simulink model "SimulationModel_FLC2"  (R2018a)
settings: Solver=ode4  StartTime=0.0  StopTime=inf  RelTol=1e-3
PreLoadFcn:
  | addLibrariesInPath('sim')
PostLoadFcn:
  | loadRobotParameters
StartFcn:
  | simApp = SimDisplay.getInstance;
  | simApp.reset;
  | simApp.TrackView.setup(double(SitesPositions), ObstaclesPositions,ObstaclesVertices,ObstaclesEdges);
values from neighbouring files (symbols this model uses):
  AngularSpeed = 300    [loadRobotParameters.m]
  AxleLength = 16.7    [loadRobotParameters.m]
  DISTANCE_APPROACH = 45    [loadRobotParameters.m]
  DISTANCE_MAX = 200    [loadRobotParameters.m]
  DISTANCE_PARKING = 10    [loadRobotParameters.m]
  do_one_run = true    [loadRobotParameters.m]
  EncL_init = 0    [loadRobotParameters.m]
  EncR_init = 0    [loadRobotParameters.m]
  EncRes = 636    [loadRobotParameters.m]
  lcam = [21, 90]    [loadRobotParameters.m]
  motorL = [-967.207000 -900.359000 -783.375000 -618.344000 -325.884000 -0.000000 0.000000 325.884000 618.344000 783.375000 900.359000 967.207000 ]    [loadRobotParameters.m]
  motorR = [-937.961000 -850.223000 -768.752000 -618.344000 -302.905000 -0.000000 0.000000 302.905000 618.344000 768.752000 850.223000 937.961000 ]    [loadRobotParameters.m]
  motorX = [-100.000000 -90.000000 -70.000000 -50.000000 -30.000000 -27.000000 27.000000 30.000000 50.000000 70.000000 90.000000 100.000000 ]    [loadRobotParameters.m]
  pcam = [24, 100]    [loadRobotParameters.m]
  RADIUS_TARGET = 5    [loadRobotParameters.m]
  S_ROT = 10    [loadRobotParameters.m]
  SPEED_APPROACH = 15    [loadRobotParameters.m]
  SPEED_BACK = 5    [loadRobotParameters.m]
  SPEED_NORMAL = 30    [loadRobotParameters.m]
  startPos = single([150 150])    [loadRobotParameters.m]
  TauMotor = 0.1    [loadRobotParameters.m]
  TH1 = 5    [loadRobotParameters.m]
  TH2 = 15    [loadRobotParameters.m]
  theta0 = 0    [loadRobotParameters.m]
  Ts = 0.1    [loadRobotParameters.m]
  WAIT_TIME = 4    [loadRobotParameters.m]
  WheelRadius = 7/2    (= 3.5)    [loadRobotParameters.m]
undefined symbols (not defined in the file or in its folder): ObstaclesEdges, ObstaclesVertices, SitesPositions
libraries: simulink_extras x2, simulink x2, Fuzzy_Type2_Lib x1, realtime_pacer_lib x1, cstblocks x1
(part 1 of 2)
CloseFcn:
  | delete(SimDisplay.getInstance());
settings Model: PauseTimes=14  NumberOfSteps=3  ExtModeTrigDuration=2  Creator=gpacitti  LastModifiedBy=root
settings DataIOCC: LimitDataPoints=on  SaveFormat=Array
settings OptimizationCC: BlockReduction=off  BooleanDataType=off  LifeSpan=inf
settings DebuggingCC: SaveWithParameterizedLinksMsg=none  SignalResolutionControl=TryResolveAllWithWarning  ParameterPrecisionLossMsg=none  AllowSymbolicDim=off  SFUnexpectedBacktrackingDiag=warning  SFNoUnconditionalDefaultTransitionDiag=warning  SFExecutionAtInitializationDiag=none
settings HardwareCC: ProdBitPerPointer=32  ProdBitPerSizeT=32  ProdBitPerPtrDiffT=32  ProdLargestAtomicFloat=None  ProdIntDivRoundTo=Undefined  ProdEndianess=Unspecified  ProdWordSize=32  ProdHWDeviceType=32-bit Generic  TargetUnknown=on
settings ModelReferenceCC: PropagateSignalLabelsOutOfModel=off
settings CodeAppCC: StateflowObjectComments=on
settings GRTTargetCC: TargetLangStandard=C89/C90 (ANSI)  GeneratePreprocessorConditionals=Disable all
settings ConfigComp: CovMetricSettings=dw  CovHtmlReporting=on  CovSaveCumulativeToWorkspaceVar=on  CovSaveSingleToWorkspaceVar=on  CovExternalEMLEnable=off  CovSFcnEnable=off
settings ConfigurationSet: Description=SimMechanics 2G

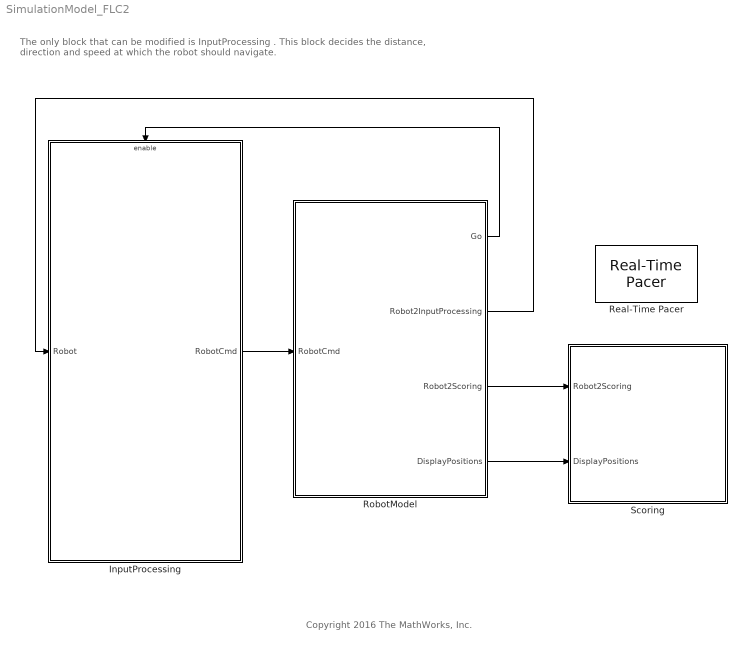
== system SimulationModel_FLC2 ==
  note: Copyright 2016 The MathWorks, Inc.
  note: The only block that can be modified is InputProcessing .
      | This block decides the distance, direction and speed at which the robot should navigate.
  InputProcessing : Subsystem
      mask Display: image('Arduino_Due_2_0274.png',[0.15,0.3,0.45,0.4]);
  Real-Time Pacer : realtime_pacer_lib/Real-Time Pacer  simTimePerRealTime=1
  RobotModel : Subsystem  mask(Robot){}
      mask help:
      | !! DO NOT MODIFY !!
      | Model representing the robot behavior including physical representation and sensors.
      |
      | Version 2.1
      mask Display: image('robot_3d.jpg',[0.4,0.7,0.45,0.25]);
  Scoring : Subsystem  mask(Scoring){}
      mask help:
      | !! DO NOT MODIFY !!
      | Model representing the judge and visualisation.
  wires:
  RobotModel/2(Robot2InputProcessing) -> InputProcessing/1(Robot)
  RobotModel/3(Robot2Scoring) -> Scoring/1(Robot2Scoring)
  RobotModel/1(Go) -> InputProcessing/Enable
  RobotModel/4(DisplayPositions) -> Scoring/2(DisplayPositions)
  InputProcessing/1(RobotCmd) -> RobotModel/1(RobotCmd)

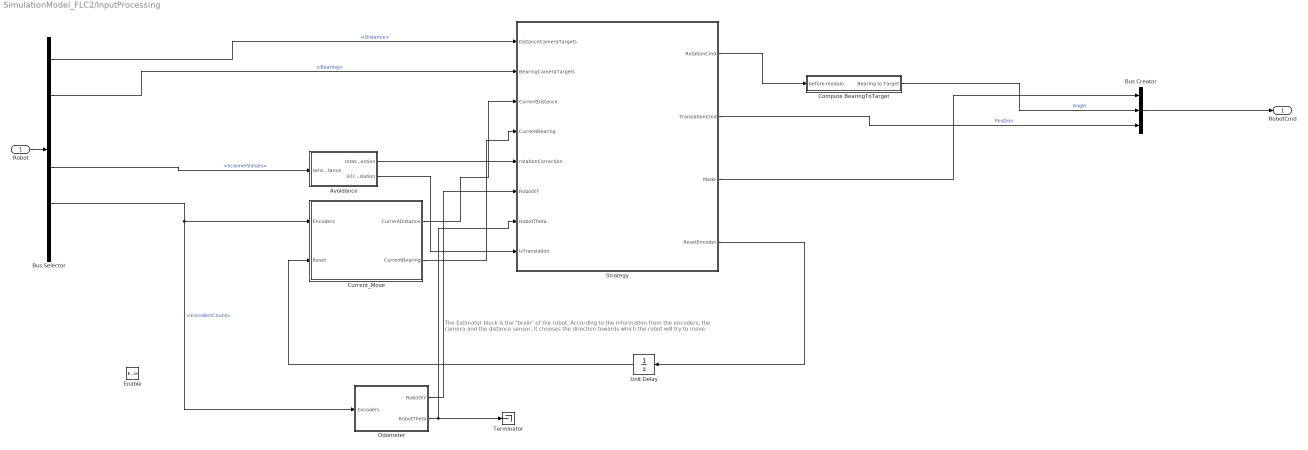
== system SimulationModel_FLC2/InputProcessing ==
  note: The Estimator block is the "brain" of the robot. According to the information from the encoders, the camera and the
      | distance sensor, it chooses the direction towards which the robot will try to move.
  Robot : Inport  OutDataTypeStr=Bus: bus_Robot
  Enable : EnablePort
  Avoidance : Subsystem
  Bus Creator : BusCreator  Inputs=3  OutDataTypeStr=Bus: bus_Command  NonVirtualBus=on
  Bus Selector : BusSelector  OutputSignals=Distance,Bearing,ScannerStatus,ScannerValues,EncodersCount,Remaining
  Compute BearingToTarget : Subsystem
  Current_Move : Subsystem
  Odometer : Subsystem
  Strategy : Stateflow chart  TreatAsAtomicUnit=on
  Terminator : Terminator
  Unit Delay : UnitDelay  SampleTime=-1
  RobotCmd : Outport  OutDataTypeStr=Bus: bus_Command
  wires:
  Robot/1 -> Bus Selector/1
  Bus Selector/2 -> Strategy/2(BearingCameraTargets)  "<Bearing>"
  Bus Selector/4 -> Avoidance/1(sensors distance)  "<ScannerValues>"
  Bus Selector/5 -> Odometer/1(Encoders), Current_Move/1(Encoders)  "<EncodersCount>"
  Bus Selector/1 -> Strategy/1(DistanceCameraTargets)  "<Distance>"
  Strategy/4(ResetEncoder) -> Unit Delay/1
  Unit Delay/1 -> Current_Move/2(Reset)
  Current_Move/1(CurrentDistance) -> Strategy/3(CurrentDistance)
  Odometer/2(RobotTheta) -> Terminator/1, Strategy/7(RobotTheta)
  Odometer/1(RobotXY) -> Strategy/6(RobotXY)
  Current_Move/2(CurrentBearing) -> Strategy/4(CurrentBearing)
  Avoidance/1(rotationCorrection) -> Strategy/5(rotationCorrection)
  Avoidance/2(isTranslation) -> Strategy/8(isTranslation)
  Strategy/1(RotationCmd) -> Compute BearingToTarget/1(before modulo)
  Bus Creator/1 -> RobotCmd/1
  Compute BearingToTarget/1(Bearing to Target) -> Bus Creator/2  "Angle"
  Strategy/2(TranslationCmd) -> Bus Creator/3  "Position"
  Strategy/3(Mode) -> Bus Creator/1

== system SimulationModel_FLC2/RobotModel ==
  RobotCmd : Inport  SampleTime=0
  Bus Creator : BusCreator  Inputs=6  OutDataTypeStr=Bus: bus_Robot  NonVirtualBus=on
  Controller : Subsystem
  Robot : Subsystem
  estimate_position : Subsystem
  Go : Outport
  Robot2InputProcessing : Outport  Port=2  OutDataTypeStr=Bus: bus_Robot
  Robot2Scoring : Outport  Port=3
  DisplayPositions : Outport  Port=4
  wires:
  Robot/6(Go) -> Go/1
  Robot/7(Robot2Scoring) -> Robot2Scoring/1
  Robot/5(ScannerValues) -> Bus Creator/5
  Robot/4(ScannerStatus) -> Bus Creator/4
  Robot/3(Bearing) -> Bus Creator/3
  Robot/2(Distance) -> Bus Creator/2
  Controller/1(MotorDemand) -> Robot/1(MotorDemand)
  Robot/1(EncoderCount) -> Bus Creator/1, estimate_position/1(Encoders), Controller/1(Encoders)
  estimate_position/1(RobotXY) -> DisplayPositions/1
  Controller/2(RemainingAngleDistance) -> Bus Creator/6  "Remaining"
  RobotCmd/1 -> Controller/2(RobotCmd)
  Bus Creator/1 -> Robot2InputProcessing/1  "Robot"

== system SimulationModel_FLC2/Scoring ==
  Robot2Scoring : Inport
  DisplayPositions : Inport  Port=2
  Bus Selector : BusSelector  OutputSignals=Position,Go
  Bus Selector1 : BusSelector  OutputSignals=LocatedTargets,RobotAngle,ArmAngleEstimated
  FigureOutput : Subsystem  TreatAsAtomicUnit=on  SimViewingDevice=on
  Referee : Subsystem
      mask Display: % image(imread('referee.png'))
  wires:
  Referee/1(Targets Located) -> FigureOutput/2(Targets Found)  "TargetsLocated"
  Referee/2(Time Last Target Found) -> FigureOutput/3(Time Last Found)  "TimeLastTargetFound"
  Referee/3(Elapsed Time_sec) -> FigureOutput/4(Time Elapsed)  "ElapsedTime"
  DisplayPositions/1 -> FigureOutput/9(DisplayPositions)
  Robot2Scoring/1 -> Bus Selector1/1, Bus Selector/1
  Bus Selector/2 -> Referee/2(Start Flag)  "<Go>"
  Bus Selector/1 -> FigureOutput/1(Position), Referee/1(Robot Position_m)  "<Position>"
  Bus Selector1/1 -> FigureOutput/5(locatedTargets)  "<LocatedTargets>"
  Bus Selector1/2 -> FigureOutput/6(robottheta)  "<RobotAngle>"
  Bus Selector1/3 -> FigureOutput/8(ArmAngleCommand), FigureOutput/7(ArmAngleEstimated)  "<ArmAngleEstimated>"

== system SimulationModel_FLC2/InputProcessing/Avoidance ==
  sensors distance : Inport
  Constant : Constant  Value=85
  Demux : Demux  Outputs=3
  Demux1 : Demux  Outputs=2
  Interval Type-2 Fuzzy Logic Controller with TR selection : Fuzzy_Type2_Lib/Interval Type-2 Fuzzy Logic Controller with TR selection  t2fisSim=t2fis_Avoidance  TRtype=0
      settings: SourceProductName=Interval Type-2 Fuzzy Logic Systems Toolbox
  Mux : Mux  Inputs=5
  Switch : Switch  Criteria=u2 > Threshold  Threshold=-1
  To File : ToFile  Filename=Avoidance.mat  MatrixName=Avoid
  rotationCorrection : Outport
  isTranslation : Outport  Port=2
  wires:
  Demux1/1 -> Mux/1, rotationCorrection/1  "rot"
  Demux1/2 -> Mux/2, isTranslation/1  "tran"
  Switch/1 -> Interval Type-2 Fuzzy Logic Controller with TR selection/1, Demux/1
  Constant/1 -> Switch/3
  sensors distance/1 -> Switch/2, Switch/1
  Mux/1 -> To File/1
  Demux/1 -> Mux/3
  Demux/2 -> Mux/4
  Demux/3 -> Mux/5
  Interval Type-2 Fuzzy Logic Controller with TR selection/1 -> Demux1/1

== system SimulationModel_FLC2/InputProcessing/Compute BearingToTarget ==
  before modulo : Inport
  Constant : Constant  Value=180  OutDataTypeStr=Inherit: Inherit via back propagation
  Constant1 : Constant  Value=360  OutDataTypeStr=Inherit: Inherit via back propagation
  Math Function1 : Math  Operator=mod  SaturateOnIntegerOverflow=on
  Sum10 : Sum  Inputs=-+|
  Sum7 : Sum  Inputs=++|
  Bearing to Target : Outport  SampleTime=Ts
  wires:
  Constant/1 -> Sum7/1, Sum10/1
  Sum7/1 -> Math Function1/1
  Constant1/1 -> Math Function1/2
  Math Function1/1 -> Sum10/2
  Sum10/1 -> Bearing to Target/1
  before modulo/1 -> Sum7/2

== system SimulationModel_FLC2/InputProcessing/Current_Move ==
  Encoders : Inport
  Reset : Inport  Port=2
  Add : Sum
  Add1 : Sum  Inputs=-+
  Demux : Demux  Outputs=2
  Gain : Gain  Gain=1/2
  Gain1 : Gain  Gain=180/(AxleLength*pi)
  d : Subsystem
  CurrentDistance : Outport
  CurrentBearing : Outport  Port=2
  wires:
  Reset/1 -> d/2(reset)
  Demux/2 -> Add/2, Add1/2
  Add1/1 -> Gain1/1
  Gain1/1 -> CurrentBearing/1
  Gain/1 -> CurrentDistance/1
  Demux/1 -> Add1/1, Add/1
  Add/1 -> Gain/1
  Encoders/1 -> d/1(encoder)
  d/1(d) -> Demux/1

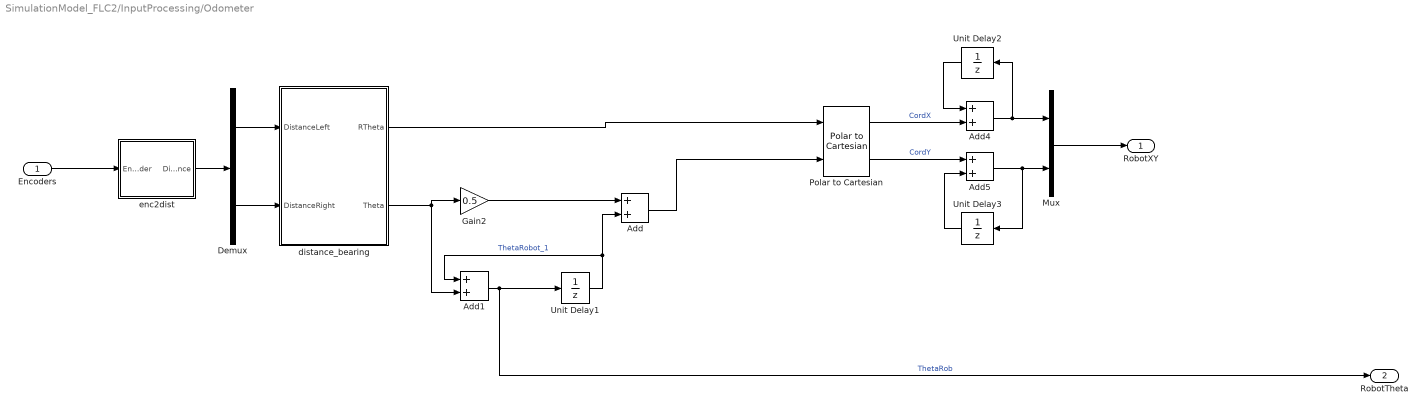
== system SimulationModel_FLC2/InputProcessing/Odometer ==
  Encoders : Inport
  Add{,1,4..5} (4 alike) : Sum
  Demux : Demux  Outputs=2
  Gain2 : Gain  Gain=0.5
  Mux : Mux  Inputs=2
  Polar to Cartesian : simulink_extras/Transformations/Polar to Cartesian
      settings: SourceProductName=Simulink  SourceProductBaseCode=SL
  Unit Delay1 : UnitDelay  DialogController=Simulink.DDGSource  InitialCondition=theta0*pi/180  SampleTime=-1
  Unit Delay2 : UnitDelay  DialogController=Simulink.DDGSource  InitialCondition=single(startPos(1))  SampleTime=-1
  Unit Delay3 : UnitDelay  DialogController=Simulink.DDGSource  InitialCondition=single(startPos(2))  SampleTime=-1
  distance_bearing : Subsystem
  enc2dist : Subsystem
  RobotXY : Outport
  RobotTheta : Outport  Port=2
  wires:
  Gain2/1 -> Add/1
  Polar to Cartesian/1 -> Add4/2  "CordX"
  Polar to Cartesian/2 -> Add5/1  "CordY"
  Add4/1 -> Unit Delay2/1, Mux/1
  Unit Delay2/1 -> Add4/1
  Add5/1 -> Mux/2, Unit Delay3/1
  Unit Delay3/1 -> Add5/2
  distance_bearing/2(Theta) -> Gain2/1, Add1/2
  Unit Delay1/1 -> Add1/1, Add/2  "ThetaRobot_1"
  Add/1 -> Polar to Cartesian/2
  Add1/1 -> RobotTheta/1, Unit Delay1/1  "ThetaRob"
  distance_bearing/1(RTheta) -> Polar to Cartesian/1
  Mux/1 -> RobotXY/1
  enc2dist/1(Distance) -> Demux/1
  Demux/1 -> distance_bearing/1(DistanceLeft)
  Demux/2 -> distance_bearing/2(DistanceRight)
  Encoders/1 -> enc2dist/1(Encoder)

== system SimulationModel_FLC2/RobotModel/Controller ==
  Encoders : Inport
  RobotCmd : Inport  Port=2  OutDataTypeStr=Bus: bus_Command
  Command2Demand : Subsystem
  FeedbackController : Subsystem  VariantControl=variantBasic
  MotorDemand : Outport  SampleTime=Ts  OutputWhenDisabled=reset  InitialOutput=0
  RemainingAngleDistance : Outport  Port=2  OutputWhenDisabled=reset  InitialOutput=0
  wires:
  FeedbackController/3(RemainingAngleDistance) -> RemainingAngleDistance/1
  FeedbackController/1(DifferentialCommand) -> Command2Demand/1(DifferentialCommand)
  FeedbackController/2(ForwardCommand) -> Command2Demand/2(ForwardCommand)
  Command2Demand/1(MotorDemand) -> MotorDemand/1
  Encoders/1 -> FeedbackController/1(Encoders)
  RobotCmd/1 -> FeedbackController/2(Cmd)

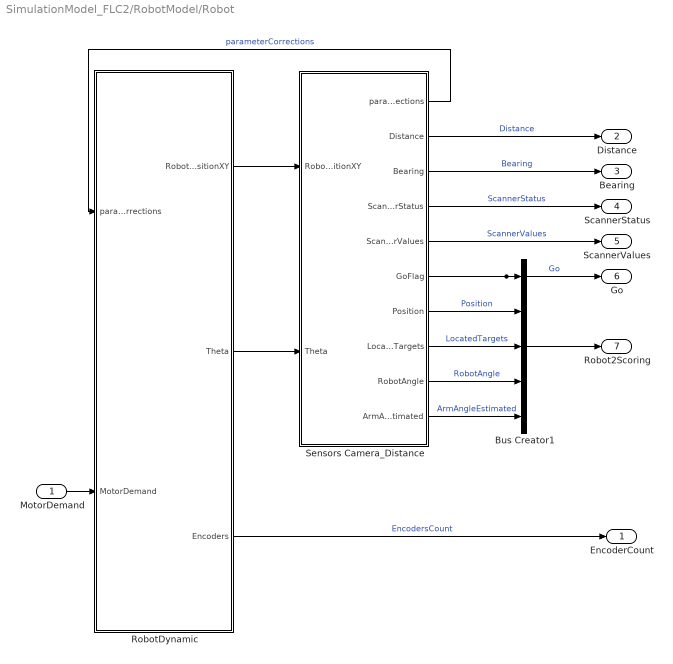
== system SimulationModel_FLC2/RobotModel/Robot ==
  MotorDemand : Inport
  Bus Creator1 : BusCreator  Inputs=5
  RobotDynamic : Subsystem
  Sensors Camera_Distance : Subsystem
  EncoderCount : Outport
  Distance : Outport  Port=2
  Bearing : Outport  Port=3
  ScannerStatus : Outport  Port=4
  ScannerValues : Outport  Port=5
  Go : Outport  Port=6
  Robot2Scoring : Outport  Port=7
  wires:
  Bus Creator1/1 -> Robot2Scoring/1
  Sensors Camera_Distance/10(ArmAngleEstimated) -> Bus Creator1/5  "ArmAngleEstimated"
  Sensors Camera_Distance/9(RobotAngle) -> Bus Creator1/4  "RobotAngle"
  Sensors Camera_Distance/7(Position) -> Bus Creator1/2  "Position"
  Sensors Camera_Distance/8(LocatedTargets) -> Bus Creator1/3  "LocatedTargets"
  MotorDemand/1 -> RobotDynamic/2(MotorDemand)
  Sensors Camera_Distance/6(GoFlag) -> Go/1, Bus Creator1/1  "Go"
  Sensors Camera_Distance/1(parameterCorrections) -> RobotDynamic/1(parameterCorrections)  "parameterCorrections"
  Sensors Camera_Distance/2(Distance) -> Distance/1  "Distance"
  Sensors Camera_Distance/3(Bearing) -> Bearing/1  "Bearing"
  Sensors Camera_Distance/4(ScannerStatus) -> ScannerStatus/1  "ScannerStatus"
  Sensors Camera_Distance/5(ScannerValues) -> ScannerValues/1  "ScannerValues"
  RobotDynamic/3(Encoders) -> EncoderCount/1  "EncodersCount"
  RobotDynamic/1(RobotPositionXY) -> Sensors Camera_Distance/1(RobotPositionXY)
  RobotDynamic/2(Theta) -> Sensors Camera_Distance/2(Theta)

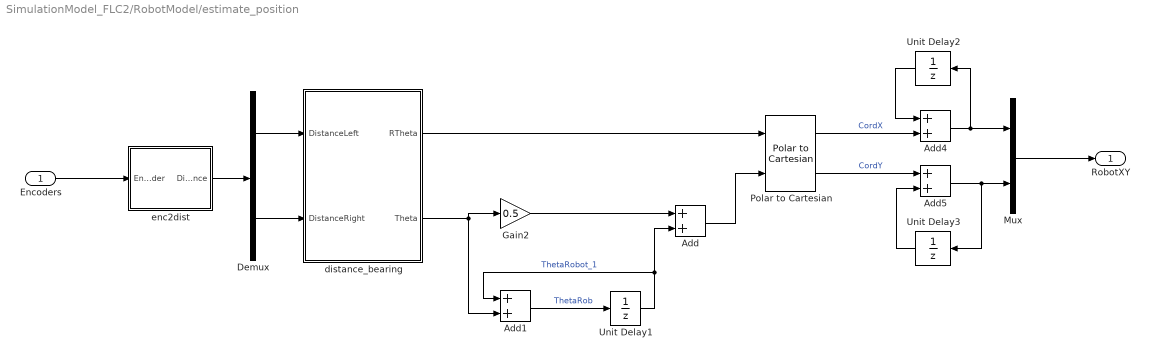
== system SimulationModel_FLC2/RobotModel/estimate_position ==
  Encoders : Inport
  Add{,1,4..5} (4 alike) : Sum
  Demux : Demux  Outputs=2
  Gain2 : Gain  Gain=0.5
  Mux : Mux  Inputs=2
  Polar to Cartesian : simulink_extras/Transformations/Polar to Cartesian
      settings: SourceProductName=Simulink  SourceProductBaseCode=SL
  Unit Delay1 : UnitDelay  DialogController=Simulink.DDGSource  InitialCondition=theta0*pi/180  SampleTime=-1
  Unit Delay2 : UnitDelay  DialogController=Simulink.DDGSource  InitialCondition=single(startPos(1))  SampleTime=-1
  Unit Delay3 : UnitDelay  DialogController=Simulink.DDGSource  InitialCondition=single(startPos(2))  SampleTime=-1
  distance_bearing : Subsystem
  enc2dist : Subsystem
  RobotXY : Outport
  wires:
  Encoders/1 -> enc2dist/1(Encoder)
  Demux/2 -> distance_bearing/2(DistanceRight)
  Demux/1 -> distance_bearing/1(DistanceLeft)
  enc2dist/1(Distance) -> Demux/1
  Mux/1 -> RobotXY/1
  distance_bearing/1(RTheta) -> Polar to Cartesian/1
  Add1/1 -> Unit Delay1/1  "ThetaRob"
  Add/1 -> Polar to Cartesian/2
  Unit Delay1/1 -> Add/2, Add1/1  "ThetaRobot_1"
  distance_bearing/2(Theta) -> Add1/2, Gain2/1
  Unit Delay3/1 -> Add5/2
  Add5/1 -> Unit Delay3/1, Mux/2
  Unit Delay2/1 -> Add4/1
  Add4/1 -> Mux/1, Unit Delay2/1
  Polar to Cartesian/2 -> Add5/1  "CordY"
  Polar to Cartesian/1 -> Add4/2  "CordX"
  Gain2/1 -> Add/1

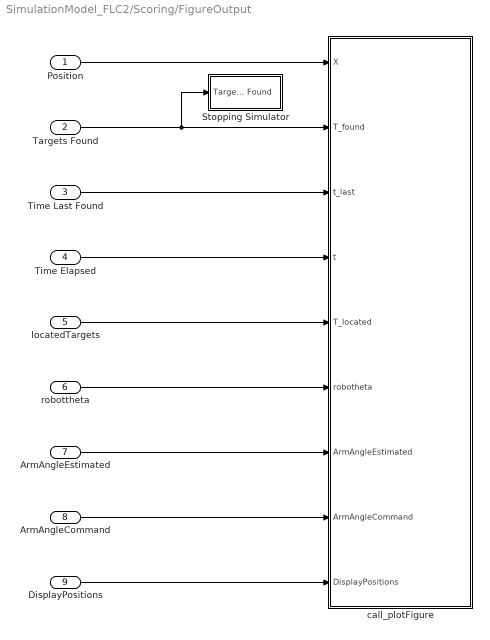
== system SimulationModel_FLC2/Scoring/FigureOutput ==
  Position : Inport
  Targets Found : Inport  Port=2
  Time Last Found : Inport  Port=3
  Time Elapsed : Inport  Port=4
  locatedTargets : Inport  Port=5
  robottheta : Inport  Port=6
  ArmAngleEstimated : Inport  Port=7
  ArmAngleCommand : Inport  Port=8
  DisplayPositions : Inport  Port=9
  Stopping Simulator : Subsystem
  call_plotFigure : MATLAB Function  TreatAsAtomicUnit=on
  wires:
  Position/1 -> call_plotFigure/1(X)
  Targets Found/1 -> Stopping Simulator/1(Targets Found), call_plotFigure/2(T_found)
  Time Last Found/1 -> call_plotFigure/3(t_last)
  Time Elapsed/1 -> call_plotFigure/4(t)
  locatedTargets/1 -> call_plotFigure/5(T_located)
  robottheta/1 -> call_plotFigure/6(robotheta)
  DisplayPositions/1 -> call_plotFigure/9(DisplayPositions)
  ArmAngleEstimated/1 -> call_plotFigure/7(ArmAngleEstimated)
  ArmAngleCommand/1 -> call_plotFigure/8(ArmAngleCommand)

== system SimulationModel_FLC2/Scoring/Referee ==
  Robot Position_m : Inport  SampleTime=Ts
  Start Flag : Inport  Port=2  OutDataTypeStr=boolean  SampleTime=Ts
  Digital Clock1 : DigitalClock  SampleTime=Ts
  Referee : Stateflow chart  TreatAsAtomicUnit=on
  Reshape : Reshape  OutputDimensionality=Row vector (2-D)
  Targets Located : Outport
  Time Last Target Found : Outport  Port=2  PortDimensions=1
  Elapsed Time_sec : Outport  Port=3  PortDimensions=1
  wires:
  Referee/1(timeLastTargetFound) -> Time Last Target Found/1
  Referee/3(targetsFound) -> Targets Located/1
  Robot Position_m/1 -> Reshape/1
  Start Flag/1 -> Referee/2(StartFlag)
  Reshape/1 -> Referee/1(robotPosition)
  Referee/2(elapsedTime) -> Elapsed Time_sec/1
  Digital Clock1/1 -> Referee/3(sim_time)

== system SimulationModel_FLC2/InputProcessing/Current_Move/d ==
  encoder : Inport
  reset : Inport  Port=2
  Add : Sum  Inputs=-+  OutDataTypeStr=single
  Gain : Gain  Gain=2*pi/EncRes
  Product : Product
  Triggered Subsystem : Subsystem  TreatAsAtomicUnit=on
  WheelRadius : Constant  Value=WheelRadius  OutDataTypeStr=Inherit: Inherit via back propagation
  d : Outport
  wires:
  Triggered Subsystem/1(encoderTarget) -> Add/1
  reset/1 -> Triggered Subsystem/Trigger
  encoder/1 -> Triggered Subsystem/1(encoderIn), Add/2
  Gain/1 -> d/1
  Add/1 -> Product/2
  Product/1 -> Gain/1
  WheelRadius/1 -> Product/1

== system SimulationModel_FLC2/InputProcessing/Odometer/distance_bearing ==
  DistanceLeft : Inport
  DistanceRight : Inport  Port=2
  Add : Sum
  Add1 : Sum  Inputs=-+
  Gain : Gain  Gain=0.5
  Gain1 : Gain  Gain=1/AxleLength
  RTheta : Outport
  Theta : Outport  Port=2
  wires:
  Gain1/1 -> Theta/1
  Add/1 -> Gain/1
  Gain/1 -> RTheta/1
  Add1/1 -> Gain1/1
  DistanceLeft/1 -> Add1/1, Add/1
  DistanceRight/1 -> Add/2, Add1/2

== system SimulationModel_FLC2/InputProcessing/Odometer/enc2dist ==
  Encoder : Inport
  Add2 : Sum  Inputs=-+
  Gain : Gain  Gain=2*pi/EncRes  OutDataTypeStr=single
  Product : Product
  Unit Delay : UnitDelay  DialogController=Simulink.DDGSource  SampleTime=-1
  WheelRadius : Constant  Value=WheelRadius  OutDataTypeStr=single
  Distance : Outport
  wires:
  Product/1 -> Gain/1
  Encoder/1 -> Product/1
  Gain/1 -> Unit Delay/1, Add2/2
  Unit Delay/1 -> Add2/1
  Add2/1 -> Distance/1
  WheelRadius/1 -> Product/2

== system SimulationModel_FLC2/RobotModel/Controller/Command2Demand ==
  DifferentialCommand : Inport
  ForwardCommand : Inport  Port=2
  Mux : Mux  Inputs=2
  Saturation : Saturate  UpperLimit=100  LowerLimit=-100
  Saturation1 : Saturate  UpperLimit=100  LowerLimit=-100
  Sum : Sum  Inputs=|++
  Sum1 : Sum  Inputs=-+|
  MotorDemand : Outport
  wires:
  Mux/1 -> MotorDemand/1
  Saturation1/1 -> Mux/2  "RightMotorDemand"
  Saturation/1 -> Mux/1  "LeftMotorDemand"
  Sum1/1 -> Saturation1/1
  Sum/1 -> Saturation/1
  ForwardCommand/1 -> Sum/1, Sum1/2  "ForwardCommand"
  DifferentialCommand/1 -> Sum/2, Sum1/1  "DifferentialCommand"

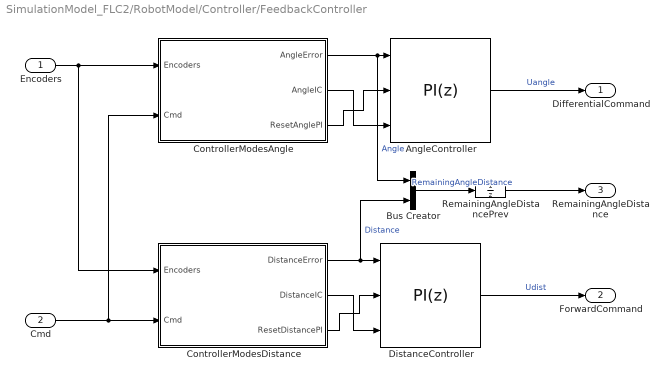
== system SimulationModel_FLC2/RobotModel/Controller/FeedbackController ==
  Encoders : Inport
  Cmd : Inport  Port=2  OutDataTypeStr=Bus: bus_Command
  AngleController : simulink/Continuous/PID Controller  Controller=PI  TimeDomain=Discrete-time  SampleTime=Ts  IntegratorMethod=Forward Euler  FilterMethod=Forward Euler  Form=Parallel  UseFilter=on  ControllerParametersSource=internal  P=1.5  I=1.5  D=1.77054210521092  N=39.6000406506001  InitialConditionSource=external  InitialConditionForIntegrator=0  InitialConditionForFilter=0  ExternalReset=either  LimitOutput=on  UpperSaturationLimit=100  LowerSaturationLimit=-100  LinearizeAsGain=off  AntiWindupMode=clamping  Kb=1  TrackingMode=off  Kt=1  PParamMin=[]  PParamMax=[]  IParamMin=[]  IParamMax=[]  DParamMin=[]  DParamMax=[]  NParamMin=[]  NParamMax=[]  KbParamMin=[]  KbParamMax=[]  KtParamMin=[]  KtParamMax=[]  POutMin=[]  POutMax=[]  IOutMin=[]  IOutMax=[]  DOutMin=[]  DOutMax=[]  NOutMin=[]  NOutMax=[]  KbOutMin=[]  KbOutMax=[]  KtOutMin=[]  KtOutMax=[]  IntegratorOutMin=[]  IntegratorOutMax=[]  FilterOutMin=[]  FilterOutMax=[]  SumOutMin=[]  SumOutMax=[]  SumI1OutMin=[]  SumI1OutMax=[]  SumI2OutMin=[]  SumI2OutMax=[]  SumI3OutMin=[]  SumI3OutMax=[]  SumDOutMin=[]  SumDOutMax=[]  SaturationOutMin=[]  SaturationOutMax=[]  IntegratorContinuousStateAttributes=''  IntegratorStateMustResolveToSignalObject=off  IntegratorRTWStateStorageClass=Auto  FilterContinuousStateAttributes=''  FilterStateMustResolveToSignalObject=off  FilterRTWStateStorageClass=Auto  DifferentiatorICPrevScaledInput=0  DifferentiatorOutMin=[]  DifferentiatorOutMax=[]  FilterDiffOutCoefMin=[]  FilterDiffOutCoefMax=[]  SumDenOutMin=[]  SumDenOutMax=[]  SumNumOutMin=[]  SumNumOutMax=[]  ReciprocalOutMin=[]  ReciprocalOutMax=[]  DivideOutMin=[]  DivideOutMax=[]  TunerSelectOption=Transfer Function Based (PID Tuner App)
  Bus Creator : BusCreator  Inputs=2  OutDataTypeStr=Bus: bus_RemainingPosition  NonVirtualBus=on
  ControllerModesAngle : Stateflow chart  TreatAsAtomicUnit=on
  ControllerModesDistance : Stateflow chart  TreatAsAtomicUnit=on
  DistanceController : simulink/Continuous/PID Controller  Controller=PI  TimeDomain=Discrete-time  SampleTime=Ts  IntegratorMethod=Forward Euler  FilterMethod=Forward Euler  Form=Parallel  UseFilter=on  ControllerParametersSource=internal  P=1.2  I=0.6  D=-10.1274478197245  N=40.1053905161445  InitialConditionSource=external  InitialConditionForIntegrator=0  InitialConditionForFilter=0  ExternalReset=either  LimitOutput=on  UpperSaturationLimit=80  LowerSaturationLimit=-80  LinearizeAsGain=off  AntiWindupMode=clamping  Kb=1  TrackingMode=off  Kt=1  PParamMin=[]  PParamMax=[]  IParamMin=[]  IParamMax=[]  DParamMin=[]  DParamMax=[]  NParamMin=[]  NParamMax=[]  KbParamMin=[]  KbParamMax=[]  KtParamMin=[]  KtParamMax=[]  POutMin=[]  POutMax=[]  IOutMin=[]  IOutMax=[]  DOutMin=[]  DOutMax=[]  NOutMin=[]  NOutMax=[]  KbOutMin=[]  KbOutMax=[]  KtOutMin=[]  KtOutMax=[]  IntegratorOutMin=[]  IntegratorOutMax=[]  FilterOutMin=[]  FilterOutMax=[]  SumOutMin=[]  SumOutMax=[]  SumI1OutMin=[]  SumI1OutMax=[]  SumI2OutMin=[]  SumI2OutMax=[]  SumI3OutMin=[]  SumI3OutMax=[]  SumDOutMin=[]  SumDOutMax=[]  SaturationOutMin=[]  SaturationOutMax=[]  IntegratorContinuousStateAttributes=''  IntegratorStateMustResolveToSignalObject=off  IntegratorRTWStateStorageClass=Auto  FilterContinuousStateAttributes=''  FilterStateMustResolveToSignalObject=off  FilterRTWStateStorageClass=Auto  DifferentiatorICPrevScaledInput=0  DifferentiatorOutMin=[]  DifferentiatorOutMax=[]  FilterDiffOutCoefMin=[]  FilterDiffOutCoefMax=[]  SumDenOutMin=[]  SumDenOutMax=[]  SumNumOutMin=[]  SumNumOutMax=[]  ReciprocalOutMin=[]  ReciprocalOutMax=[]  DivideOutMin=[]  DivideOutMax=[]  TunerSelectOption=Transfer Function Based (PID Tuner App)
  RemainingAngleDistancePrev : UnitDelay  SampleTime=-1
  DifferentialCommand : Outport
  ForwardCommand : Outport  Port=2
  RemainingAngleDistance : Outport  Port=3  OutDataTypeStr=Bus: bus_RemainingPosition
  wires:
  ControllerModesAngle/1(AngleError) -> AngleController/1, Bus Creator/1  "Angle"
  ControllerModesDistance/3(ResetDistancePI) -> DistanceController/2
  ControllerModesDistance/2(DistanceIC) -> DistanceController/3
  ControllerModesDistance/1(DistanceError) -> DistanceController/1, Bus Creator/2  "Distance"
  ControllerModesAngle/3(ResetAnglePI) -> AngleController/2
  ControllerModesAngle/2(AngleIC) -> AngleController/3
  AngleController/1 -> DifferentialCommand/1  "Uangle"
  RemainingAngleDistancePrev/1 -> RemainingAngleDistance/1
  Bus Creator/1 -> RemainingAngleDistancePrev/1  "RemainingAngleDistance"
  Cmd/1 -> ControllerModesDistance/2(Cmd), ControllerModesAngle/2(Cmd)
  Encoders/1 -> ControllerModesDistance/1(Encoders), ControllerModesAngle/1(Encoders)
  DistanceController/1 -> ForwardCommand/1  "Udist"

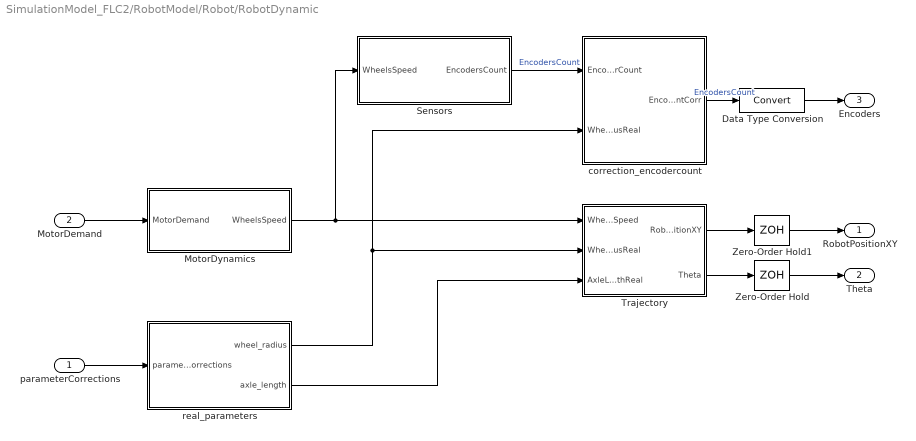
== system SimulationModel_FLC2/RobotModel/Robot/RobotDynamic ==
  parameterCorrections : Inport
  MotorDemand : Inport  Port=2
  Data Type Conversion : DataTypeConversion
  MotorDynamics : Subsystem
  Sensors : Subsystem
  Trajectory : Subsystem
  Zero-Order Hold : ZeroOrderHold  SampleTime=Ts
  Zero-Order Hold1 : ZeroOrderHold  SampleTime=Ts
  correction_encodercount : Subsystem
  real_parameters : Subsystem
  RobotPositionXY : Outport
  Theta : Outport  Port=2
  Encoders : Outport  Port=3
  wires:
  Data Type Conversion/1 -> Encoders/1
  real_parameters/1(wheel_radius) -> correction_encodercount/2(WheelRadiusReal), Trajectory/2(WheelsRadiusReal)
  real_parameters/2(axle_length) -> Trajectory/3(AxleLengthReal)
  Sensors/1(EncodersCount) -> correction_encodercount/1(EncoderCount)  "EncodersCount"
  parameterCorrections/1 -> real_parameters/1(parameterCorrections)
  Zero-Order Hold/1 -> Theta/1
  Zero-Order Hold1/1 -> RobotPositionXY/1
  Trajectory/2(Theta) -> Zero-Order Hold/1
  Trajectory/1(RobotPositionXY) -> Zero-Order Hold1/1
  correction_encodercount/1(EncoderCountCorr) -> Data Type Conversion/1  "EncodersCount"
  MotorDemand/1 -> MotorDynamics/1(MotorDemand)
  MotorDynamics/1(WheelsSpeed) -> Trajectory/1(WheelsSpeed), Sensors/1(WheelsSpeed)

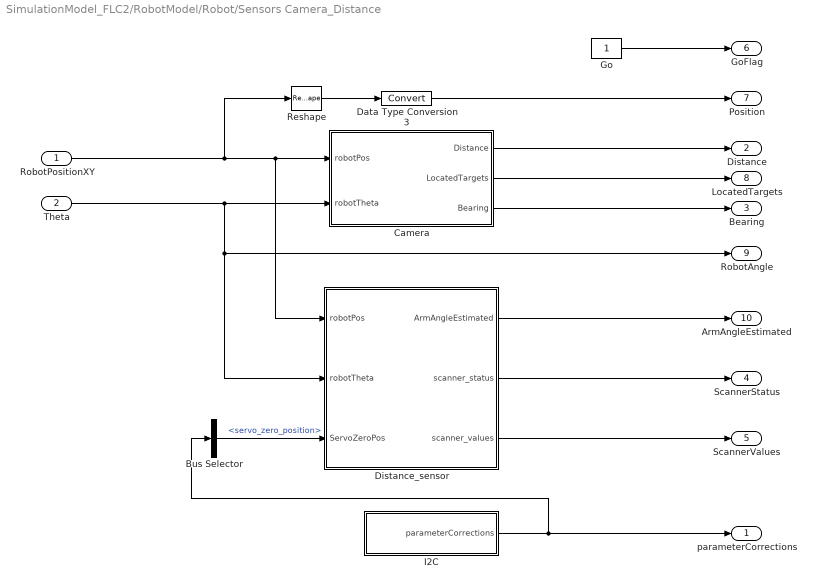
== system SimulationModel_FLC2/RobotModel/Robot/Sensors Camera_Distance ==
  RobotPositionXY : Inport
  Theta : Inport  Port=2
  Bus Selector : BusSelector  OutputSignals=servo_zero_position
  Camera : Subsystem
  Data Type Conversion3 : DataTypeConversion
  Distance_sensor : Subsystem
  Go : Constant  OutMin=0  OutMax=1  OutDataTypeStr=boolean  SampleTime=0.1
  I2C : Subsystem
  Reshape : Reshape  OutputDimensionality=Row vector (2-D)
  parameterCorrections : Outport
  Distance : Outport  Port=2  OutDataTypeStr=int16
  Bearing : Outport  Port=3  OutDataTypeStr=int8
  ScannerStatus : Outport  Port=4
  ScannerValues : Outport  Port=5
  GoFlag : Outport  Port=6
  Position : Outport  Port=7
  LocatedTargets : Outport  Port=8
  RobotAngle : Outport  Port=9
  ArmAngleEstimated : Outport  Port=10
  wires:
  Go/1 -> GoFlag/1
  Bus Selector/1 -> Distance_sensor/3(ServoZeroPos)  "<servo_zero_position>"
  I2C/1(parameterCorrections) -> parameterCorrections/1, Bus Selector/1
  Distance_sensor/3(scanner_values) -> ScannerValues/1
  Distance_sensor/2(scanner_status) -> ScannerStatus/1
  Distance_sensor/1(ArmAngleEstimated) -> ArmAngleEstimated/1
  Camera/3(Bearing) -> Bearing/1
  Camera/2(LocatedTargets) -> LocatedTargets/1
  Camera/1(Distance) -> Distance/1
  Theta/1 -> Camera/2(robotTheta), Distance_sensor/2(robotTheta), RobotAngle/1
  RobotPositionXY/1 -> Reshape/1, Camera/1(robotPos), Distance_sensor/1(robotPos)
  Reshape/1 -> Data Type Conversion3/1
  Data Type Conversion3/1 -> Position/1

== system SimulationModel_FLC2/RobotModel/estimate_position/distance_bearing ==
  DistanceLeft : Inport
  DistanceRight : Inport  Port=2
  Add : Sum
  Add1 : Sum  Inputs=-+
  Gain : Gain  Gain=0.5
  Gain1 : Gain  Gain=1/AxleLength
  RTheta : Outport
  Theta : Outport  Port=2
  wires:
  DistanceRight/1 -> Add1/2, Add/2
  DistanceLeft/1 -> Add/1, Add1/1
  Add1/1 -> Gain1/1
  Gain/1 -> RTheta/1
  Add/1 -> Gain/1
  Gain1/1 -> Theta/1

== system SimulationModel_FLC2/RobotModel/estimate_position/enc2dist ==
  Encoder : Inport
  Add2 : Sum  Inputs=-+
  Gain : Gain  Gain=2*pi/EncRes  OutDataTypeStr=single
  Product : Product
  Unit Delay : UnitDelay  DialogController=Simulink.DDGSource  SampleTime=-1
  WheelRadius : Constant  Value=WheelRadius  OutDataTypeStr=single
  Distance : Outport
  wires:
  WheelRadius/1 -> Product/2
  Add2/1 -> Distance/1
  Unit Delay/1 -> Add2/1
  Gain/1 -> Add2/2, Unit Delay/1
  Encoder/1 -> Product/1
  Product/1 -> Gain/1

== system SimulationModel_FLC2/Scoring/FigureOutput/Stopping Simulator ==
  Targets Found : Inport
  Constant : Constant  Value=do_one_run
  Data Type Conversion : DataTypeConversion  OutDataTypeStr=double
  Logical Operator1 : Logic  AllPortsSameDT=off  OutDataTypeStr=boolean
  MinMax : MinMax
  Stop Simulation : Stop
  wires:
  Targets Found/1 -> Data Type Conversion/1
  Data Type Conversion/1 -> MinMax/1
  MinMax/1 -> Logical Operator1/1
  Constant/1 -> Logical Operator1/2
  Logical Operator1/1 -> Stop Simulation/1

== system SimulationModel_FLC2/InputProcessing/Current_Move/d/Triggered Subsystem ==
  encoderIn : Inport
  Trigger : TriggerPort  TriggerType=either  VariantControl=(inherit)
  encoderTarget : Outport
  wires:
  encoderIn/1 -> encoderTarget/1

== system SimulationModel_FLC2/RobotModel/Controller/FeedbackController/ControllerModesAngle/CurrentMove.CurrentMoveFcn ==
  enc : Inport  OutDataTypeStr=int32  PortDimensions=2
  zero : Inport  Port=2  OutDataTypeStr=int32  PortDimensions=2
  f : TriggerPort  TriggerType=function-call  VariantControl=(inherit)
      settings: CopyFcn=Stateflow.SLINSF.SimulinkMan.removeBlockPreDeleteFcn  PreDeleteFcn=Stateflow.SLINSF.SimulinkMan.unsafePredeleteFcn
  Add : Sum  Inputs=+-  OutDataTypeStr=single
  CountToRad : Gain  Gain=2*pi/EncRes
  Demux : Demux  Outputs=2
  Gain : Gain  Gain=WheelRadius/AxleLength
  Rad2Deg : Gain  Gain=rad2deg(1)
  Sum2 : Sum  Inputs=+-
  angle : Outport
  wires:
  zero/1 -> Add/2
  enc/1 -> Add/1
  Gain/1 -> Rad2Deg/1
  Sum2/1 -> Gain/1
  Demux/1 -> Sum2/1
  Demux/2 -> Sum2/2
  CountToRad/1 -> Demux/1
  Rad2Deg/1 -> angle/1  "theta"
  Add/1 -> CountToRad/1

== system SimulationModel_FLC2/RobotModel/Controller/FeedbackController/ControllerModesAngle/ModeControl.errorFactor ==
  pos : Inport  OutDataTypeStr=single  PortDimensions=1
  f : TriggerPort  TriggerType=function-call  VariantControl=(inherit)
      settings: CopyFcn=Stateflow.SLINSF.SimulinkMan.removeBlockPreDeleteFcn  PreDeleteFcn=Stateflow.SLINSF.SimulinkMan.unsafePredeleteFcn
  1-D Lookup Table : Lookup_n-D  NumberOfTableDimensions=1  BreakpointsForDimension1=[10;20;40;60;80;100]  Table=[60;10;25;20;10;10]  ExtrapMethod=Clip  InternalRulePriority=Speed  RndMeth=Simplest  InputSameDT=on
  Bias : Bias  Bias=1
  Divide : Product  Inputs=*/
  factor : Outport  OutDataTypeStr=single  PortDimensions=1
  wires:
  1-D Lookup Table/1 -> Divide/2
  pos/1 -> Divide/1, 1-D Lookup Table/1
  Divide/1 -> Bias/1
  Bias/1 -> factor/1

== system SimulationModel_FLC2/RobotModel/Controller/FeedbackController/ControllerModesDistance/CurrentMove.CurrentMoveFcn ==
  enc : Inport  OutDataTypeStr=int32  PortDimensions=2
  zero : Inport  Port=2  OutDataTypeStr=int32  PortDimensions=2
  f : TriggerPort  TriggerType=function-call  VariantControl=(inherit)
      settings: CopyFcn=Stateflow.SLINSF.SimulinkMan.removeBlockPreDeleteFcn  PreDeleteFcn=Stateflow.SLINSF.SimulinkMan.unsafePredeleteFcn
  Add : Sum  Inputs=+-  OutDataTypeStr=single
  CountToRad : Gain  Gain=2*pi/EncRes
  Demux : Demux  Outputs=2
  Gain1 : Gain  Gain=0.5*WheelRadius
  Sum4 : Sum
  distance : Outport
  wires:
  Add/1 -> CountToRad/1
  Gain1/1 -> distance/1  "distance"
  CountToRad/1 -> Demux/1
  Demux/2 -> Sum4/2
  Demux/1 -> Sum4/1
  Sum4/1 -> Gain1/1
  enc/1 -> Add/1
  zero/1 -> Add/2

== system SimulationModel_FLC2/RobotModel/Robot/RobotDynamic/MotorDynamics ==
  MotorDemand : Inport
  Demux : Demux  Outputs=2
  Dynamics : cstblocks/LTI System  sys=tf(1,[TauMotor 1])*eye(2)  IC=[]
  Left_motor_table : Lookup_n-D  NumberOfTableDimensions=1  BreakpointsForDimension1=motorX  Table=motorL  ExtrapMethod=Clip  InternalRulePriority=Speed  OutDataTypeStr=Inherit: Inherit via back propagation  RndMeth=Simplest  InputSameDT=on
  Mux1 : Mux  Inputs=2
  Right_motor_table : Lookup_n-D  NumberOfTableDimensions=1  BreakpointsForDimension1=motorX  Table=motorR  ExtrapMethod=Clip  InternalRulePriority=Speed  OutDataTypeStr=Inherit: Inherit via back propagation  RndMeth=Simplest  InputSameDT=on
  WheelsSpeed : Outport  PortDimensions=2
  wires:
  MotorDemand/1 -> Demux/1
  Demux/2 -> Right_motor_table/1
  Demux/1 -> Left_motor_table/1
  Mux1/1 -> Dynamics/1  "Speed Demand d°/s"
  Left_motor_table/1 -> Mux1/1
  Right_motor_table/1 -> Mux1/2
  Dynamics/1 -> WheelsSpeed/1  "Wheels Velocity d°/s"

== system SimulationModel_FLC2/RobotModel/Robot/RobotDynamic/Sensors ==
  WheelsSpeed : Inport
  Encoder Quantization : Quantizer  QuantizationInterval=(360/EncRes)
  Encoder Reading : ZeroOrderHold  SampleTime=Ts
  angular_position : Integrator  InitialCondition=[EncL_init;EncR_init]
  deg2encoderCount : Gain  Gain=EncRes/360  OutDataTypeStr=Inherit: Inherit via back propagation
  EncodersCount : Outport
  wires:
  deg2encoderCount/1 -> Encoder Reading/1
  Encoder Quantization/1 -> EncodersCount/1
  angular_position/1 -> deg2encoderCount/1  "WheelsPosition d°"
  Encoder Reading/1 -> Encoder Quantization/1
  WheelsSpeed/1 -> angular_position/1  "Wheels Velocity d°/s"

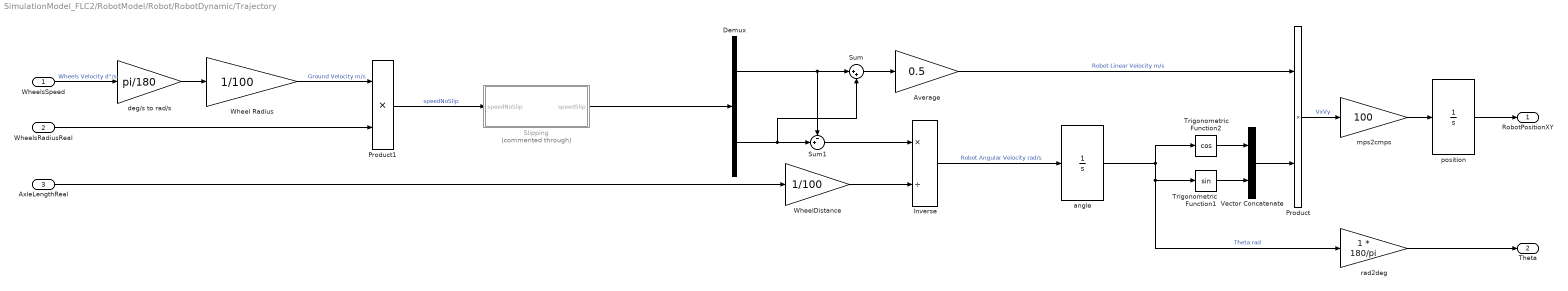
== system SimulationModel_FLC2/RobotModel/Robot/RobotDynamic/Trajectory ==
  WheelsSpeed : Inport  PortDimensions=2
  WheelsRadiusReal : Inport  Port=2  PortDimensions=2
  AxleLengthReal : Inport  Port=3  PortDimensions=1
  Average : Gain  Gain=0.5
  Demux : Demux  Outputs=2
  Inverse : Product  Inputs=*/
  Product : Product
  Product1 : Product
  Slipping : Subsystem  Commented=through
  Sum : Sum  Inputs=|++
  Sum1 : Sum  Inputs=-+|
  Trigonometric Function1 : Trigonometry
  Trigonometric Function2 : Trigonometry  Operator=cos
  Vector Concatenate : Concatenate
  Wheel Radius : Gain  Gain=1/100
  WheelDistance : Gain  Gain=1/100
  angle : Integrator  InitialCondition=theta0 * pi/180
  deg/s to rad/s : Gain  Gain=pi/180
  mps2cmps : Gain  Gain=100
  position : Integrator  InitialCondition=double(startPos)
  rad2deg : Gain  Gain=1 * 180/pi
  RobotPositionXY : Outport
  Theta : Outport  Port=2
  wires:
  Slipping/1(speedSlip) -> Demux/1
  Product1/1 -> Slipping/1(speedNoSlip)  "speedNoSlip"
  WheelDistance/1 -> Inverse/2
  WheelsRadiusReal/1 -> Product1/2
  Wheel Radius/1 -> Product1/1  "Ground Velocity m/s"
  AxleLengthReal/1 -> WheelDistance/1
  WheelsSpeed/1 -> deg/s to rad/s/1  "Wheels Velocity d°/s"
  rad2deg/1 -> Theta/1
  position/1 -> RobotPositionXY/1
  mps2cmps/1 -> position/1
  deg/s to rad/s/1 -> Wheel Radius/1
  Inverse/1 -> angle/1  "Robot Angular Velocity rad/s"
  Product/1 -> mps2cmps/1  "VxVy"
  Sum1/1 -> Inverse/1
  Demux/1 -> Sum/1, Sum1/1
  Demux/2 -> Sum/2, Sum1/2
  Sum/1 -> Average/1
  Average/1 -> Product/1  "Robot Linear Velocity m/s"
  Vector Concatenate/1 -> Product/2
  Trigonometric Function1/1 -> Vector Concatenate/2
  Trigonometric Function2/1 -> Vector Concatenate/1
  angle/1 -> Trigonometric Function2/1, Trigonometric Function1/1, rad2deg/1  "Theta rad"

== system SimulationModel_FLC2/RobotModel/Robot/RobotDynamic/correction_encodercount ==
  EncoderCount : Inport
  WheelRadiusReal : Inport  Port=2
  Divide : Product  Inputs=*/
  Product : Product
  WheelRadius : Constant  Value=WheelRadius
  EncoderCountCorr : Outport
  wires:
  WheelRadiusReal/1 -> Divide/2
  Product/1 -> EncoderCountCorr/1  "corrected"
  EncoderCount/1 -> Product/1  "measured"
  Divide/1 -> Product/2  "corr_factor"
  WheelRadius/1 -> Divide/1  "wheelRadius_ideal"

== system SimulationModel_FLC2/RobotModel/Robot/RobotDynamic/real_parameters ==
  parameterCorrections : Inport
  Add : Sum
  Add1 : Sum
  AxleLength : Constant  Value=AxleLength
  Bus Selector : BusSelector  OutputSignals=wheel_left_radius,wheel_right_radius
  Bus Selector1 : BusSelector  OutputSignals=axle_length
  Mux : Mux  Inputs=2
  WheelRadius : Constant  Value=WheelRadius
  wheel_radius : Outport
  axle_length : Outport  Port=2
  wires:
  Add1/1 -> axle_length/1
  AxleLength/1 -> Add1/1
  Bus Selector1/1 -> Add1/2  "<axle_length>"
  Mux/1 -> Add/2
  Bus Selector/2 -> Mux/2  "<wheel_right_radius>"
  Bus Selector/1 -> Mux/1  "<wheel_left_radius>"
  parameterCorrections/1 -> Bus Selector/1, Bus Selector1/1
  WheelRadius/1 -> Add/1
  Add/1 -> wheel_radius/1

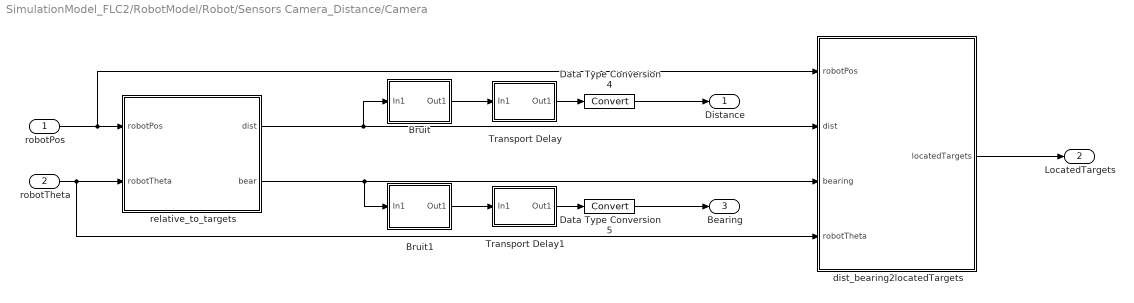
== system SimulationModel_FLC2/RobotModel/Robot/Sensors Camera_Distance/Camera ==
  robotPos : Inport
  robotTheta : Inport  Port=2
  Bruit : Subsystem
  Bruit1 : Subsystem
  Data Type Conversion4 : DataTypeConversion
  Data Type Conversion5 : DataTypeConversion
  Transport Delay : Subsystem  mask{timeDelay=0.300, initialOutput=zeros(size(6,1),1), initialBufferSize=1024, useFixedBufferSize=off, directFeedthoughOfInputDuringLinearization=off, padeOrder=0}
      mask prompts: initialOutput "Initial output"; initialBufferSize "Initial buffer size"; useFixedBufferSize "Use fixed buffer size"; directFeedthoughOfInputDuringLinearization "Direct feedthough of input during linearization"; padeOrder "Pade order (for linearization):"
  Transport Delay1 : Subsystem  mask{timeDelay=0.300, initialOutput=zeros(size(6,1),1), initialBufferSize=1024, useFixedBufferSize=off, directFeedthoughOfInputDuringLinearization=off, padeOrder=0}
      mask prompts: initialOutput "Initial output"; initialBufferSize "Initial buffer size"; useFixedBufferSize "Use fixed buffer size"; directFeedthoughOfInputDuringLinearization "Direct feedthough of input during linearization"; padeOrder "Pade order (for linearization):"
  dist_bearing2locatedTargets : MATLAB Function  TreatAsAtomicUnit=on
  relative_to_targets : MATLAB Function  TreatAsAtomicUnit=on
  Distance : Outport  OutDataTypeStr=int16
  LocatedTargets : Outport  Port=2
  Bearing : Outport  Port=3  OutDataTypeStr=int8
  wires:
  robotPos/1 -> relative_to_targets/1(robotPos), dist_bearing2locatedTargets/1(robotPos)
  robotTheta/1 -> relative_to_targets/2(robotTheta), dist_bearing2locatedTargets/4(robotTheta)
  Data Type Conversion5/1 -> Bearing/1
  Bruit/1(Out1) -> Transport Delay/1(In1)
  relative_to_targets/1(dist) -> dist_bearing2locatedTargets/2(dist), Bruit/1(In1)
  Bruit1/1(Out1) -> Transport Delay1/1(In1)
  Transport Delay1/1(Out1) -> Data Type Conversion5/1
  dist_bearing2locatedTargets/1(locatedTargets) -> LocatedTargets/1
  relative_to_targets/2(bear) -> dist_bearing2locatedTargets/3(bearing), Bruit1/1(In1)
  Data Type Conversion4/1 -> Distance/1
  Transport Delay/1(Out1) -> Data Type Conversion4/1

== system SimulationModel_FLC2/RobotModel/Robot/Sensors Camera_Distance/Distance_sensor ==
  robotPos : Inport  SampleTime=Ts
  robotTheta : Inport  Port=2  SampleTime=Ts
  ServoZeroPos : Inport  Port=3  SampleTime=Ts
  ArmAngleEstimator : Subsystem
  Scanner : Stateflow chart  TreatAsAtomicUnit=on
  arm_distance : MATLAB Function  TreatAsAtomicUnit=on
  ArmAngleEstimated : Outport
  scanner_status : Outport  Port=2
  scanner_values : Outport  Port=3
  wires:
  Scanner/1(scanner_status) -> scanner_status/1
  Scanner/2(scanner_value) -> scanner_values/1
  arm_distance/1(armDist) -> Scanner/1(ArmDist)
  Scanner/3(ArmAngle) -> ArmAngleEstimator/2("  ArmAngleCommand")
  robotPos/1 -> arm_distance/1(robotPos)
  robotTheta/1 -> arm_distance/2(robotTheta)
  ArmAngleEstimator/1(ArmAngleEstimated) -> ArmAngleEstimated/1, arm_distance/3(armAngle)
  ServoZeroPos/1 -> ArmAngleEstimator/1("  ServoZeroPos")

== system SimulationModel_FLC2/RobotModel/Robot/Sensors Camera_Distance/I2C ==
  Bus Creator : BusCreator  Inputs=6
  axle_length : Constant  Value=0  OutDataTypeStr=Inherit: Inherit via back propagation
  motor_left_deadband : Constant  Value=0  OutDataTypeStr=Inherit: Inherit via back propagation
  motor_right_deadband : Constant  Value=0  OutDataTypeStr=Inherit: Inherit via back propagation
  servo_zero_position : Constant  Value=0  OutDataTypeStr=Inherit: Inherit via back propagation
  wheel_left_radius : Constant  Value=0  OutDataTypeStr=Inherit: Inherit via back propagation
  wheel_right_radius : Constant  Value=0  OutDataTypeStr=Inherit: Inherit via back propagation
  parameterCorrections : Outport
  wires:
  axle_length/1 -> Bus Creator/6  "axle_length"
  servo_zero_position/1 -> Bus Creator/5  "servo_zero_position"
  wheel_right_radius/1 -> Bus Creator/2  "wheel_right_radius"
  motor_left_deadband/1 -> Bus Creator/3  "motor_left_deadband"
  motor_right_deadband/1 -> Bus Creator/4  "motor_right_deadband"
  Bus Creator/1 -> parameterCorrections/1
  wheel_left_radius/1 -> Bus Creator/1  "wheel_left_radius"

== system SimulationModel_FLC2/RobotModel/Robot/RobotDynamic/Trajectory/Slipping ==
  speedNoSlip : Inport
  Abs : Abs
  Product2 : Product
  Rate Limiter : RateLimiter  RisingSlewLimit=[1 1]*3  FallingSlewLimit=-1000  SampleTimeMode=inherited
  Sign : Signum
  speedSlip : Outport
  wires:
  speedNoSlip/1 -> Abs/1, Sign/1
  Product2/1 -> speedSlip/1  "speedSlip"
  Abs/1 -> Rate Limiter/1
  Rate Limiter/1 -> Product2/2
  Sign/1 -> Product2/1

== system SimulationModel_FLC2/RobotModel/Robot/Sensors Camera_Distance/Camera/Bruit ==
  In1 : Inport
  Add : Sum
  Data Type Conversion4 : DataTypeConversion
  Product : Product
  Uniform Random Number : UniformRandomNumber  Minimum=-0.05  Maximum=0.05  SampleTime=Ts
  Out1 : Outport
  wires:
  Add/1 -> Out1/1
  Data Type Conversion4/1 -> Product/1
  Uniform Random Number/1 -> Data Type Conversion4/1
  Product/1 -> Add/1
  In1/1 -> Product/2, Add/2

== system SimulationModel_FLC2/RobotModel/Robot/Sensors Camera_Distance/Camera/Bruit1 ==
  In1 : Inport
  Add : Sum
  Data Type Conversion4 : DataTypeConversion
  Product : Product
  Uniform Random Number : UniformRandomNumber  Minimum=-0.05  Maximum=0.05  SampleTime=Ts
  Out1 : Outport
  wires:
  Add/1 -> Out1/1
  In1/1 -> Product/2, Add/2
  Product/1 -> Add/1
  Uniform Random Number/1 -> Data Type Conversion4/1
  Data Type Conversion4/1 -> Product/1

== system SimulationModel_FLC2/RobotModel/Robot/Sensors Camera_Distance/Camera/Transport Delay ==
  In1 : Inport
  Data Type Conversion : DataTypeConversion  OutDataTypeStr=double
  Data Type Conversion4 : DataTypeConversion  OutDataTypeStr=single
  Transport Delay : TransportDelay  DelayTime=timeDelay  InitialOutput=initialOutput  BufferSize=initialBufferSize  PadeOrder=padeOrder
  Zero-Order Hold : ZeroOrderHold  SampleTime=Ts
  Out1 : Outport
  wires:
  Zero-Order Hold/1 -> Out1/1
  In1/1 -> Data Type Conversion/1
  Data Type Conversion4/1 -> Zero-Order Hold/1
  Data Type Conversion/1 -> Transport Delay/1
  Transport Delay/1 -> Data Type Conversion4/1

== system SimulationModel_FLC2/RobotModel/Robot/Sensors Camera_Distance/Camera/Transport Delay1 ==
  In1 : Inport
  Data Type Conversion : DataTypeConversion  OutDataTypeStr=double
  Data Type Conversion4 : DataTypeConversion  OutDataTypeStr=single
  Transport Delay : TransportDelay  DelayTime=timeDelay  InitialOutput=initialOutput  BufferSize=initialBufferSize  PadeOrder=padeOrder
  Zero-Order Hold : ZeroOrderHold  SampleTime=Ts
  Out1 : Outport
  wires:
  Zero-Order Hold/1 -> Out1/1
  Transport Delay/1 -> Data Type Conversion4/1
  Data Type Conversion/1 -> Transport Delay/1
  Data Type Conversion4/1 -> Zero-Order Hold/1
  In1/1 -> Data Type Conversion/1

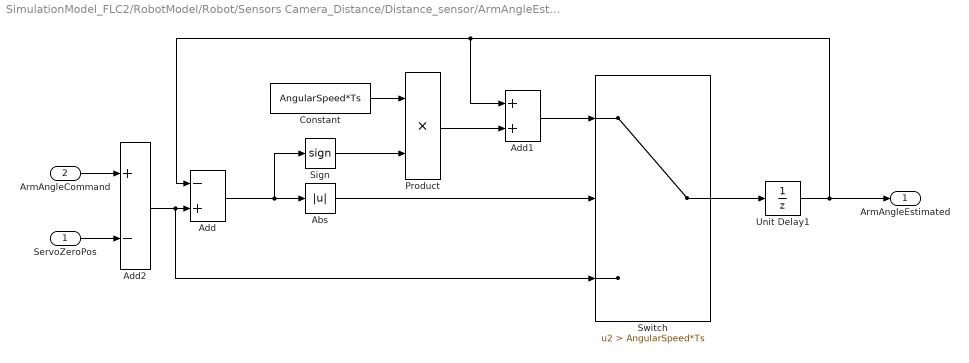
== system SimulationModel_FLC2/RobotModel/Robot/Sensors Camera_Distance/Distance_sensor/ArmAngleEstimator ==
  "  ServoZeroPos" : Inport
  "  ArmAngleCommand" : Inport  Port=2
  Abs : Abs
  Add : Sum  Inputs=-+
  Add1 : Sum
  Add2 : Sum  Inputs=+-
  Constant : Constant  Value=AngularSpeed*Ts
  Product : Product
  Sign : Signum
  Switch : Switch  Criteria=u2 > Threshold  Threshold=AngularSpeed*Ts
  Unit Delay1 : UnitDelay  DialogController=Simulink.DDGSource  SampleTime=-1
  ArmAngleEstimated : Outport
  wires:
  "  ArmAngleCommand"/1 -> Add2/1
  Add2/1 -> Add/2, Switch/3
  "  ServoZeroPos"/1 -> Add2/2
  Unit Delay1/1 -> ArmAngleEstimated/1, Add1/1, Add/1
  Add1/1 -> Switch/1
  Product/1 -> Add1/2
  Sign/1 -> Product/2
  Constant/1 -> Product/1
  Switch/1 -> Unit Delay1/1
  Abs/1 -> Switch/2
  Add/1 -> Abs/1, Sign/1

== stateflow chart SimulationModel_FLC2/RobotModel/Controller/FeedbackController/ControllerModesAngle ==
  state CurrentMove [parallel]
    settings: executionOrder=1
    state Normal
      entry:
      EncodersZero = Encoders;
      entry,during:
      CurrentAngle = CurrentMoveFcn(Encoders,EncodersZero);
    state angle = CurrentMoveFcn(enc,zero) [function]
    (default) -> Normal
    Normal -> Normal : Reset
  state ModeControl [parallel]
    settings: executionOrder=2
    state SpeedControl
      entry:
      CurrentMove.Reset;
      AngleError = Cmd.Angle;
      PrevAngle = CurrentAngle;
      during:
      AngleError = 0.08 * errorFactor(Cmd.Position) * ...
      (Cmd.Angle - (CurrentAngle-PrevAngle)/Ts);
      PrevAngle = CurrentAngle;
    state DistanceControl
      entry:
      CurrentMove.Reset;
      entry,during:
      AngleError = Cmd.Angle - CurrentAngle;
    state factor = errorFactor(pos) [function]
    (default) -> (junction 73)
    (junction 73) -> (junction 72) [order 1] : [Cmd.Mode == EMode.SPEED]
    (junction 73) -> DistanceControl [order 2]
    (junction 72) -> SpeedControl
    SpeedControl -> DistanceControl : [Cmd.Mode == EMode.DISTANCE]
    DistanceControl -> SpeedControl : [Cmd.Mode == EMode.SPEED]
  state ErrorInitialCondition [parallel]
    settings: executionOrder=3
    (default) -> (junction 178)
    ErrorInitialCondition -> (junction 178)
    (junction 178) -> (junction 168)
    (junction 168) -> (junction 169) [order 1] : [abs(AngleError) < 30 && ...
        | abs(Cmd.Position) < 1]
    (junction 168) -> (junction 167) [order 2] : {
        | AngleIC = single(0);
        | }
    (junction 169) -> (junction 172) : {
        | AngleIC = 30 * sign(Cmd.Angle) - AngleError;
        | }
    (junction 172) -> (junction 167)
    (junction 167) -> (junction 173)
  state ResetIntegrator [parallel]
    settings: executionOrder=4
    (default) -> (junction 203) : {
        | PrevCmd = Cmd.Angle;
        | PrevMode = Cmd.Mode;
        | }
    ResetIntegrator -> (junction 203)
    (junction 203) -> (junction 205) [order 1] : [Cmd.Mode ~= PrevMode]
    (junction 203) -> (junction 197) [order 2]
    (junction 205) -> (junction 198)
    (junction 197) -> (junction 198) [order 1] : [sign(Cmd.Angle) ~= sign(PrevCmd)]
    (junction 197) -> (junction 212) [order 2]
    (junction 198) -> (junction 213)
    (junction 212) -> (junction 213) [order 1] : [Cmd.Mode == EMode.SPEED && Cmd.Angle ~= PrevCmd]
    (junction 212) -> (junction 199) [order 2]
    (junction 213) -> (junction 200) : {
        | ResetAnglePI;
        | }
    (junction 200) -> (junction 199)
    (junction 199) -> (junction 201) : {
        | PrevCmd = Cmd.Angle;
        | PrevMode = Cmd.Mode;
        | }
  data: enc function_input int32 size=2; zero function_input int32 size=2; angle function_output; EncodersZero local int32 size=2; PrevAngle local; pos function_input single size=1; factor function_output single size=1; PrevCmd local; PrevMode local; Encoders input int32 size=2; CurrentAngle local single; AngleError output single size=1; Cmd input Bus: bus_Command; Ts parameter; AngleIC output
  events: Reset local FUNCTION_CALL_EVENT; ResetAnglePI output EITHER_EDGE_EVENT

== stateflow chart SimulationModel_FLC2/RobotModel/Robot/Sensors Camera_Distance/Distance_sensor/Scanner ==
  state ScanDistance
    state Scanning
      state LookFront
        entry:
        ArmAngle = int8(0);
        exit:
        scanner_value(EPosition.MIDDLE) = ArmDist;
        scanner_status = EPosition.MIDDLE;
      state LookLeft
        entry:
        ArmAngle = int8(25);
        exit:
        scanner_value(EPosition.LEFT) = ArmDist;
        scanner_status = EPosition.LEFT;
      state LookRight
        entry:
        ArmAngle = int8(-25);
        exit:
        scanner_value(EPosition.RIGHT) = ArmDist;
        scanner_status = EPosition.RIGHT;
      (default) -> LookFront : {
          | scanner_value = int8(-1*ones(1,3));
          | scanner_status = EPosition.NO;
          | }
      LookLeft -> LookFront [order 1] : after(4,tick)
      LookLeft -> LookFront [order 2] : [after(3,tick) && ArmDist == -1]
      LookFront -> LookRight [order 1] : after(3,tick)
      LookFront -> LookRight [order 2] : [after(2,tick) && ArmDist == -1]
      LookRight -> LookLeft [order 1] : after(3,tick)
      LookRight -> LookLeft [order 2] : [after(2,tick) && ArmDist == -1]
    state Idle
      entry:
      ArmAngle = int8(0);
      during,exit:
      scanner_value = int8(-1*ones(1,3));
      scanner_status = EPosition.NO;
    (default) -> Scanning
    Scanning -> Idle : pauseScanner
    Idle -> Scanning : resumeScanner
  data: ArmDist input; scanner_status output Enum: EPosition; scanner_value output int8; ArmAngle output
  events: resumeScanner local FUNCTION_CALL_EVENT; pauseScanner local FUNCTION_CALL_EVENT
